simulink model "FFT4dSpace_1"  (R2021a)
settings: Solver=ode1  StartTime=0.0  StopTime=Inf  FixedStep=Ts  RelTol=1e-5
PostLoadFcn:
  | if any(exist('dsrtsu_mdlpostloadfcn', 'file') ~= 0), dsrtsu_mdlpostloadfcn('Execute', bdroot); end
InitFcn:
  | , if any(exist('rtifpga_mdlclblib', 'file') ~= 0), rtifpga_mdlclblib('Init', bdroot); end,
  | , if any(exist('dsmpb_private', 'file') ~= 0), dsmpb_private('dsmpb_mdlclblib', 'Init', bdroot); end,
values from neighbouring files (symbols this model uses):
  Ts_1kHz = 1e-3    (= 0.001)    [FFT4dSpace_1_i.m]
undefined symbols (not defined in the file or in its folder): CalibNormed, conv, mdlPara, PWMpara, Ro1_Be2, scaleHV, supplyPressure4VPPM
libraries: dsmpblib x46, tllib x2, dspxfrm3 x1, dspsigops x1
(part 2 of 2)

== system FFT4dSpace_1/RTI Data ==
  RTI Data Store : Subsystem  Tag="struct('private',struct('version',struct('dsVer',uint32(2),'dsVerCreation',uint32(2),'RTI',struct('ver','7.12','type','RTI1202')),'access',struct('type','Model','isPerm',1,'created',['29-Oct-2019 15:07:12'],'modified',['07-Feb-2024 10:56:01'],'location','')),'public',struct('main',struct('data',[]),'sub',struct('name',{{'FFT4dSpace_1'}},'data',{{struct('TH',struct('thTaskInfo',struct('taskType',{'TIMER','HWINT','TMRINT','SWINT','GLINT'},'tasksNumOf',{2,0,0,0,0},'srcIds',{{'TIMERA','TIMERA2'},{},{},{},{}},'taskNames',{{['Timer Task 1'],['Timer Task 2']},{},{},{},{}})),'th_tc',struct('dataType',{'TASK','TASK'},'taskGroupId',{'',''},'taskGroupList',{{},{}},'taskSchedulingPolicy',{'FCFS','FCFS'},'taskType',{'TIMER','TIMER'},'blkh',{-1,-1},'srcId',{'TIMERA','TIMERA2'},'srcSgnName',{['Timer A interrupt'],['Timer Task 1']},'srcCpuName',{'',''},'taskName',{['Timer Task 1  [5e-05] s'],['Timer Task 2  [0.001] s']},'taskNameDisplayExt',{'',''},'smplTime',{5e-5,0.001},'smplTimeOffs',{0,0},'hasFixedPriority',{0,0},'priority',{1,2},'hasFixedOvc',{0,0},'ovcType',{1,1},'ovcMax',{1,1}),'tc_th',struct('dataType',{'TASK','TASK'},'taskGroupId',{'',''},'taskGroupList',{{},{}},'taskSchedulingPolicy',{'FCFS','FCFS'},'taskType',{'TIMER','TIMER'},'blkh',{-1,-1},'srcId',{'TIMERA','TIMERA2'},'srcSgnName',{['Timer A interrupt'],['Timer Task 1']},'srcCpuName',{'',''},'taskName',{['Timer Task 1  [5e-05] s'],['Timer Task 2  [0.001] s']},'taskNameDisplayExt',{'',''},'smplTime',{5e-5,0.001},'smplTimeOffs',{0,0},'hasFixedPriority',{0,0},'priority',{1,2},'hasFixedOvc',{0,0},'ovcType',{1,1},'ovcMax',{1,1}),'FSIValue','0','NISValue','1')}})))"  mask(RTI_DATA_STORE){}
      mask help:
      | RTI Data Store Block. This block is used by RTI to store internal model dependent data. Deleting this block will result in data loss.
      |
      | NEVER DELETE, COPY, OR MODIFY THIS BLOCK!
      mask Help:
      | RTI Data Store Block. This block is used by RTI to store internal model dependent data. Deleting this block will result in data loss.
      | 
      | NEVER DELETE, COPY, OR MODIFY THIS BLOCK!
      mask Display: text(0.5, 0.5, ' ', 'HorizontalAlignment', 'center');

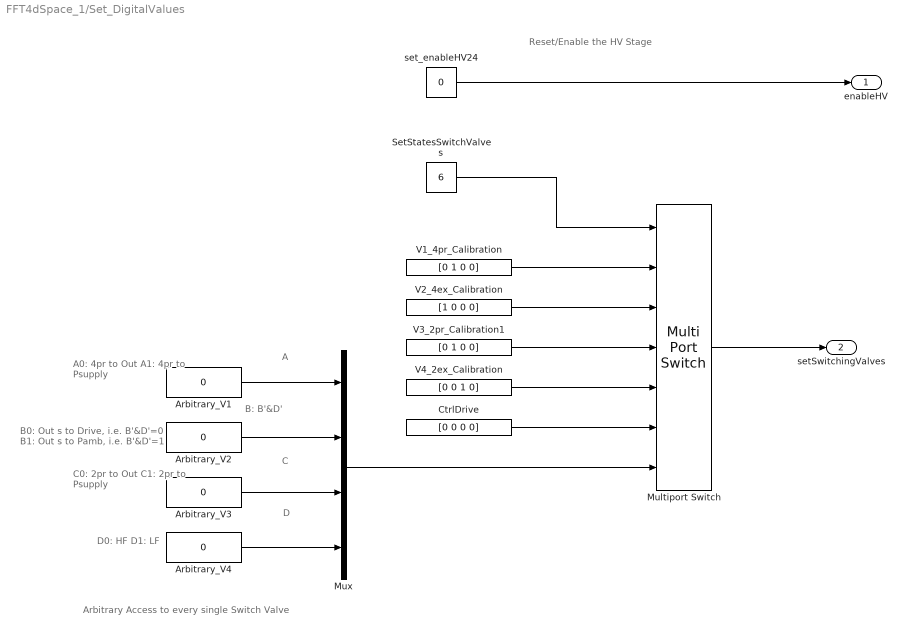
== system FFT4dSpace_1/Set_DigitalValues ==
  note: A
  note: A0: 4pr to Out
      | A1: 4pr to Psupply
  note: Arbitrary Access to every single Switch Valve
  note: Reset/Enable the HV Stage
  note: C0: 2pr to Out
      | C1: 2pr to Psupply
  note: D0: HF
      | D1: LF
  note: B0: Out s to Drive, i.e. B'&D'=0
      | B1: Out s to Pamb, i.e. B'&D'=1
  note: B: B'&D'
  note: C
  note: D
  Arbitrary_V{1..4} (4 alike) : Constant  Value=0
  CtrlDrive : Constant  Value=[0 0 0 0]  OutDataTypeStr=boolean
  Multiport Switch : MultiPortSwitch  Inputs=6
  Mux : Mux
  SetStatesSwitchValves : Constant  Value=6
  V1_4pr_Calibration : Constant  Value=[0 1 0 0]  OutDataTypeStr=boolean
  V2_4ex_Calibration : Constant  Value=[1 0 0 0]  OutDataTypeStr=boolean
  V3_2pr_Calibration1 : Constant  Value=[0 1 0 0]  OutDataTypeStr=boolean
  V4_2ex_Calibration : Constant  Value=[0 0 1 0]  OutDataTypeStr=boolean
  set_enableHV24 : Constant  Value=0  OutDataTypeStr=boolean
  "enableHV " : Outport  VectorParamsAs1DForOutWhenUnconnected=off
  setSwitchingValves : Outport  Port=2  VectorParamsAs1DForOutWhenUnconnected=off
  wires:
  SetStatesSwitchValves/1 -> Multiport Switch/1
  V1_4pr_Calibration/1 -> Multiport Switch/2
  V3_2pr_Calibration1/1 -> Multiport Switch/4
  V2_4ex_Calibration/1 -> Multiport Switch/3
  V4_2ex_Calibration/1 -> Multiport Switch/5
  CtrlDrive/1 -> Multiport Switch/6
  Mux/1 -> Multiport Switch/7
  Multiport Switch/1 -> setSwitchingValves/1
  set_enableHV24/1 -> "enableHV "/1
  Arbitrary_V2/1 -> Mux/2
  Arbitrary_V4/1 -> Mux/4
  Arbitrary_V3/1 -> Mux/3
  Arbitrary_V1/1 -> Mux/1

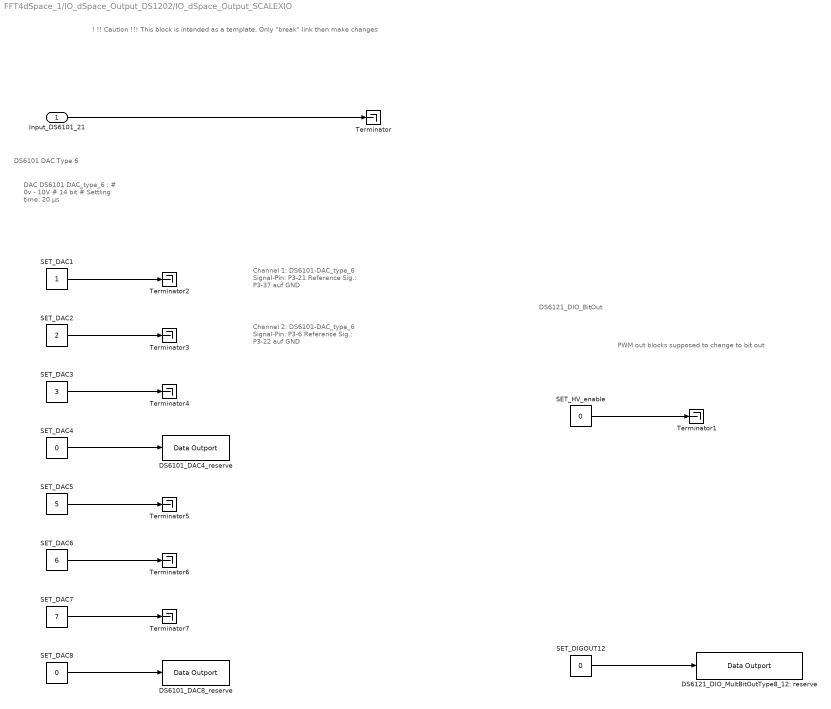
== system FFT4dSpace_1/IO_dSpace_Output_DS1202/IO_dSpace_Output_SCALEXIO ==
  note: PWM out blocks supposed to change to bit out
  note: DS6121_DIO_BitOut
  note: Channel 1: DS6101-DAC_type_6
      | Signal-Pin: P3-21
      | Reference Sig.: P3-37 auf GND
  note: DS6101 DAC Type 6
  note: Channel 2: DS6101-DAC_type_6
      | Signal-Pin: P3-6
      | Reference Sig.: P3-22 auf GND
  note: DAC DS6101 DAC_type_6 :
      | # 0v - 10V
      | # 14 bit
      | # Settling time: 20 µs
  note: ! !! Caution !!!
      | This block is intended as a template.
      | Only "break" link then make changes
  Input_DS6101_21 : Inport
  DS6101_DAC4_reserve : dsmpblib/Data Outport  Priority=-10000
      settings: SourceProductName=dSPACE Model Interface Blockset
  DS6101_DAC8_reserve : dsmpblib/Data Outport  Priority=-10000
      settings: SourceProductName=dSPACE Model Interface Blockset
  DS6121_DIO_MultBitOutType8_12: reserve : dsmpblib/Data Outport  Priority=-10000
      settings: SourceProductName=dSPACE Model Interface Blockset
  SET_DAC1 : Constant
  SET_DAC2 : Constant  Value=2
  SET_DAC3 : Constant  Value=3
  SET_DAC4 : Constant  Value=0
  SET_DAC5 : Constant  Value=5
  SET_DAC6 : Constant  Value=6
  SET_DAC7 : Constant  Value=7
  SET_DAC8 : Constant  Value=0
  SET_DIGOUT12 : Constant  Value=0  OutDataTypeStr=boolean
  SET_HV_enable : Constant  Value=0  OutDataTypeStr=boolean
  Terminator{,1..7} (8 alike) : Terminator
  wires:
  SET_DAC1/1 -> Terminator2/1
  Input_DS6101_21/1 -> Terminator/1
  SET_DAC2/1 -> Terminator3/1
  SET_DAC4/1 -> DS6101_DAC4_reserve/1
  SET_DAC3/1 -> Terminator4/1
  SET_DAC6/1 -> Terminator6/1
  SET_DAC5/1 -> Terminator5/1
  SET_DAC7/1 -> Terminator7/1
  SET_DAC8/1 -> DS6101_DAC8_reserve/1
  SET_HV_enable/1 -> Terminator1/1
  SET_DIGOUT12/1 -> DS6121_DIO_MultBitOutType8_12: reserve/1

== system FFT4dSpace_1/IO_dSpace_Output_DS1202/PWMcompNegativ ==
  In1 : Inport
  Add1 : Sum
  Constant1 : Constant  Value=0
  Constant2 : Constant  Value=PWMpara.offsetNegativ
  Switch : Switch  Criteria=u2 > Threshold  Threshold=PWMpara.thresholdNegativ
  PWMplusNegativ : Outport
  wires:
  Constant1/1 -> Switch/3
  Switch/1 -> Add1/1
  Constant2/1 -> Switch/1
  Add1/1 -> PWMplusNegativ/1  "PWMplusNegativ"
  In1/1 -> Add1/2, Switch/2

== system FFT4dSpace_1/IO_dSpace_Output_DS1202/PWMcompPositiv ==
  In1 : Inport
  Add1 : Sum
  Constant1 : Constant  Value=0
  Constant2 : Constant  Value=PWMpara.offsetPositiv
  Switch : Switch  Criteria=u2 > Threshold  Threshold=PWMpara.thresholdPositiv
  PWMplusPositiv : Outport
  wires:
  Constant1/1 -> Switch/3
  Switch/1 -> Add1/1
  Constant2/1 -> Switch/1
  Add1/1 -> PWMplusPositiv/1  "PWMplusPositiv"
  In1/1 -> Add1/2, Switch/2

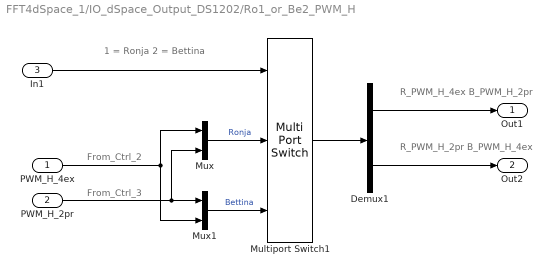
== system FFT4dSpace_1/IO_dSpace_Output_DS1202/Ro1_or_Be2_PWM_H ==
  note: 1 = Ronja
      | 2 = Bettina
  note: From_Ctrl_2
  note: R_PWM_H_4ex
      | B_PWM_H_2pr
  note: R_PWM_H_2pr
      | B_PWM_H_4ex
  note: From_Ctrl_3
  PWM_H_4ex : Inport
  PWM_H_2pr : Inport  Port=2
  In1 : Inport  Port=3
  Demux1 : Demux  Outputs=2
  Multiport Switch1 : MultiPortSwitch  Inputs=2
  Mux : Mux  Inputs=2
  Mux1 : Mux  Inputs=2
  Out1 : Outport
  Out2 : Outport  Port=2
  wires:
  Mux1/1 -> Multiport Switch1/3  "Bettina"
  Mux/1 -> Multiport Switch1/2  "Ronja"
  PWM_H_2pr/1 -> Mux/2, Mux1/1
  Multiport Switch1/1 -> Demux1/1
  Demux1/1 -> Out1/1
  PWM_H_4ex/1 -> Mux/1, Mux1/2
  Demux1/2 -> Out2/1
  In1/1 -> Multiport Switch1/1

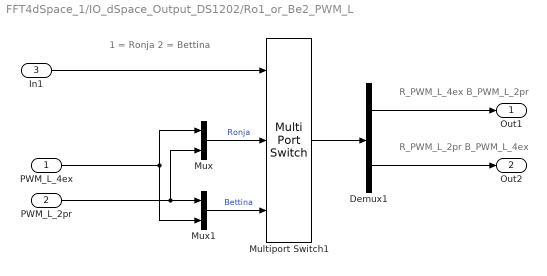
== system FFT4dSpace_1/IO_dSpace_Output_DS1202/Ro1_or_Be2_PWM_L ==
  note: R_PWM_L_4ex
      | B_PWM_L_2pr
  note: R_PWM_L_2pr
      | B_PWM_L_4ex
  note: 1 = Ronja
      | 2 = Bettina
  PWM_L_4ex : Inport
  PWM_L_2pr : Inport  Port=2
  In1 : Inport  Port=3
  Demux1 : Demux  Outputs=2
  Multiport Switch1 : MultiPortSwitch  Inputs=2
  Mux : Mux  Inputs=2
  Mux1 : Mux  Inputs=2
  Out1 : Outport
  Out2 : Outport  Port=2
  wires:
  Mux1/1 -> Multiport Switch1/3  "Bettina"
  Mux/1 -> Multiport Switch1/2  "Ronja"
  PWM_L_2pr/1 -> Mux/2, Mux1/1
  Multiport Switch1/1 -> Demux1/1
  Demux1/1 -> Out1/1
  PWM_L_4ex/1 -> Mux/1, Mux1/2
  Demux1/2 -> Out2/1
  In1/1 -> Multiport Switch1/1

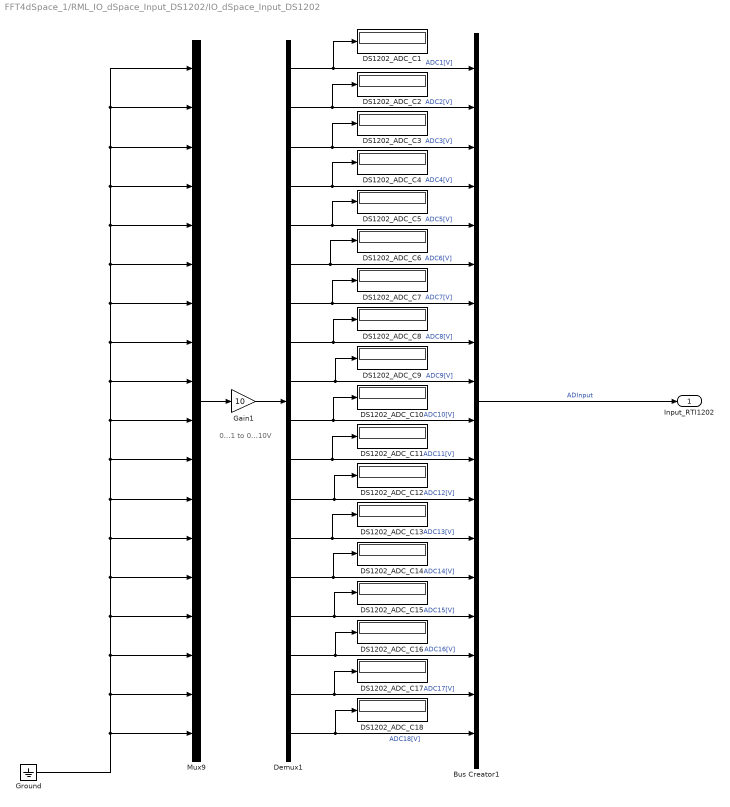
== system FFT4dSpace_1/RML_IO_dSpace_Input_DS1202/IO_dSpace_Input_DS1202 ==
  note: 0...1 to 0...10V
  Bus Creator1 : BusCreator  Inputs=18
  DS1202_ADC_C{1..18} (18 alike) : Display
  Demux1 : Demux  Outputs=18
  Gain1 : Gain  Gain=10
  Ground : Ground
  Mux9 : Mux  Inputs=18
  Input_RTI1202 : Outport
  wires:
  Gain1/1 -> Demux1/1
  Mux9/1 -> Gain1/1
  Demux1/16 -> DS1202_ADC_C16/1, Bus Creator1/16  "ADC16[V]"
  Demux1/15 -> DS1202_ADC_C15/1, Bus Creator1/15  "ADC15[V]"
  Demux1/14 -> DS1202_ADC_C14/1, Bus Creator1/14  "ADC14[V]"
  Demux1/13 -> DS1202_ADC_C13/1, Bus Creator1/13  "ADC13[V]"
  Demux1/12 -> DS1202_ADC_C12/1, Bus Creator1/12  "ADC12[V]"
  Demux1/11 -> DS1202_ADC_C11/1, Bus Creator1/11  "ADC11[V]"
  Demux1/10 -> DS1202_ADC_C10/1, Bus Creator1/10  "ADC10[V]"
  Demux1/9 -> Bus Creator1/9, DS1202_ADC_C9/1  "ADC9[V]"
  Demux1/8 -> DS1202_ADC_C8/1, Bus Creator1/8  "ADC8[V]"
  Demux1/7 -> DS1202_ADC_C7/1, Bus Creator1/7  "ADC7[V]"
  Demux1/6 -> DS1202_ADC_C6/1, Bus Creator1/6  "ADC6[V]"
  Demux1/5 -> DS1202_ADC_C5/1, Bus Creator1/5  "ADC5[V]"
  Demux1/4 -> DS1202_ADC_C4/1, Bus Creator1/4  "ADC4[V]"
  Demux1/3 -> DS1202_ADC_C3/1, Bus Creator1/3  "ADC3[V]"
  Demux1/2 -> DS1202_ADC_C2/1, Bus Creator1/2  "ADC2[V]"
  Demux1/1 -> DS1202_ADC_C1/1, Bus Creator1/1  "ADC1[V]"
  Bus Creator1/1 -> Input_RTI1202/1  "ADInput"
  Demux1/17 -> DS1202_ADC_C17/1, Bus Creator1/17  "ADC17[V]"
  Demux1/18 -> Bus Creator1/18, DS1202_ADC_C18/1  "ADC18[V]"
  Ground/1 -> Mux9/18, Mux9/17, Mux9/16, Mux9/15, Mux9/14, Mux9/13, Mux9/12, Mux9/11, Mux9/10, Mux9/9, Mux9/8, Mux9/7, Mux9/6, Mux9/5, Mux9/4, Mux9/3, Mux9/2, Mux9/1

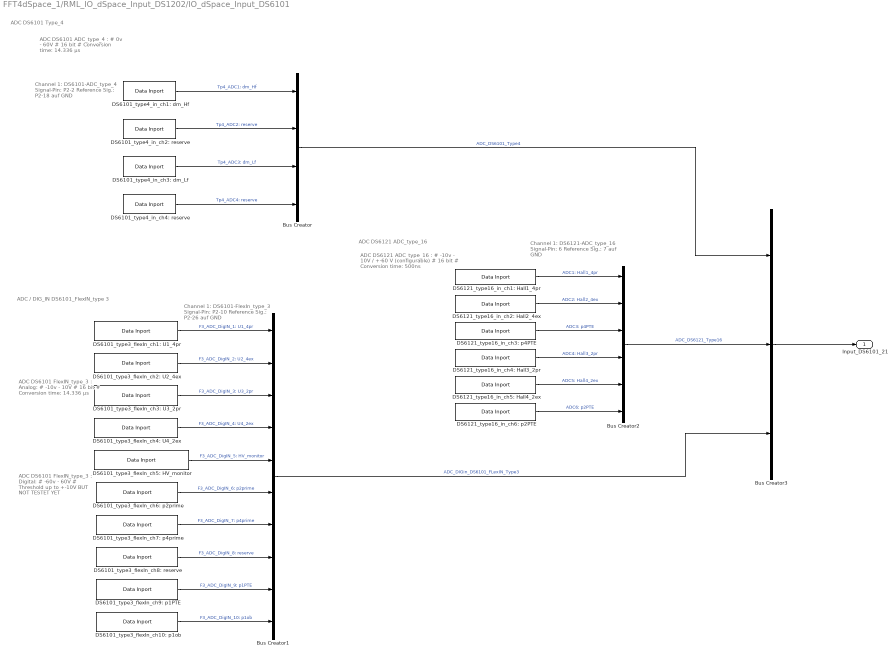
== system FFT4dSpace_1/RML_IO_dSpace_Input_DS1202/IO_dSpace_Input_DS6101 ==
  note: ADC / DIG_IN DS6101_FlexIN_type 3
  note: ADC DS6101 Type_4
  note: ADC DS6121 ADC_type_16
  note: Channel 1: DS6101-ADC_type_4
      | Signal-Pin: P2-2
      | Reference Sig.: P2-18 auf GND
  note: ADC DS6101 ADC_type_4 :
      | # 0v - 60V
      | # 16 bit
      | # Conversion time: 14.336 µs
  note: Channel 1: DS6101-FlexIn_type_3
      | Signal-Pin: P2-10
      | Reference Sig.: P2-26 auf GND
  note: ADC DS6101 FlexIN_type_3 :
      | Analog:
      | # -10v - 10V
      | # 16 bit
      | # Conversion time: 14.336 µs
  note: ADC DS6101 FlexIN_type_3 :
      | Digital:
      | # -60v - 60V
      | # Threshold up to +-10V
      |
      | BUT NOT TESTET YET
  note: Channel 1: DS6121-ADC_type_16
      | Signal-Pin: 6
      | Reference Sig.: 7 auf GND
  note: ADC DS6121 ADC_type_16 :
      | # -10v - 10V / +-60 V (configurable)
      | # 16 bit
      | # Conversion time: 500ns
  Bus Creator : BusCreator  Inputs=4
  Bus Creator1 : BusCreator  Inputs=10
  Bus Creator2 : BusCreator  Inputs=6
  Bus Creator3 : BusCreator  Inputs=3
  DS6101_type3_flexIn_ch10: p1ob : dsmpblib/Data Inport  Priority=10000
      settings: SourceProductName=dSPACE Model Interface Blockset
  DS6101_type3_flexIn_ch1: U1_4pr : dsmpblib/Data Inport  Priority=10000
      settings: SourceProductName=dSPACE Model Interface Blockset
  "DS6101_type3_flexIn_ch2: U2_4ex " : dsmpblib/Data Inport  Priority=10000
      settings: SourceProductName=dSPACE Model Interface Blockset
  DS6101_type3_flexIn_ch3: U3_2pr : dsmpblib/Data Inport  Priority=10000
      settings: SourceProductName=dSPACE Model Interface Blockset
  DS6101_type3_flexIn_ch4: U4_2ex : dsmpblib/Data Inport  Priority=10000
      settings: SourceProductName=dSPACE Model Interface Blockset
  DS6101_type3_flexIn_ch5: HV_monitor : dsmpblib/Data Inport  Priority=10000
      settings: SourceProductName=dSPACE Model Interface Blockset
  DS6101_type3_flexIn_ch6: p2prime : dsmpblib/Data Inport  Priority=10000
      settings: SourceProductName=dSPACE Model Interface Blockset
  DS6101_type3_flexIn_ch7: p4prime : dsmpblib/Data Inport  Priority=10000
      settings: SourceProductName=dSPACE Model Interface Blockset
  DS6101_type3_flexIn_ch8: reserve : dsmpblib/Data Inport  Priority=10000
      settings: SourceProductName=dSPACE Model Interface Blockset
  DS6101_type3_flexIn_ch9: p1PTE : dsmpblib/Data Inport  Priority=10000
      settings: SourceProductName=dSPACE Model Interface Blockset
  DS6101_type4_in_ch1: dm_Hf : dsmpblib/Data Inport  Priority=10000
      settings: SourceProductName=dSPACE Model Interface Blockset
  DS6101_type4_in_ch2: reserve : dsmpblib/Data Inport  Priority=10000
      settings: SourceProductName=dSPACE Model Interface Blockset
  DS6101_type4_in_ch3: dm_Lf : dsmpblib/Data Inport  Priority=10000
      settings: SourceProductName=dSPACE Model Interface Blockset
  DS6101_type4_in_ch4: reserve : dsmpblib/Data Inport  Priority=10000
      settings: SourceProductName=dSPACE Model Interface Blockset
  DS6121_type16_in_ch1: Hall1_4pr : dsmpblib/Data Inport  Priority=10000
      settings: SourceProductName=dSPACE Model Interface Blockset
  DS6121_type16_in_ch2: Hall2_4ex : dsmpblib/Data Inport  Priority=10000
      settings: SourceProductName=dSPACE Model Interface Blockset
  DS6121_type16_in_ch3: p4PTE : dsmpblib/Data Inport  Priority=10000
      settings: SourceProductName=dSPACE Model Interface Blockset
  DS6121_type16_in_ch4: Hall3_2pr : dsmpblib/Data Inport  Priority=10000
      settings: SourceProductName=dSPACE Model Interface Blockset
  DS6121_type16_in_ch5: Hall4_2ex : dsmpblib/Data Inport  Priority=10000
      settings: SourceProductName=dSPACE Model Interface Blockset
  DS6121_type16_in_ch6: p2PTE : dsmpblib/Data Inport  Priority=10000
      settings: SourceProductName=dSPACE Model Interface Blockset
  Input_DS6101_21 : Outport
  wires:
  "DS6101_type3_flexIn_ch2: U2_4ex "/1 -> Bus Creator1/2  "F3_ADC_DigIN_2: U2_4ex"
  DS6121_type16_in_ch1: Hall1_4pr/1 -> Bus Creator2/1  "ADC1: Hall1_4pr"
  DS6101_type4_in_ch1: dm_Hf/1 -> Bus Creator/1  "Tp4_ADC1: dm_Hf"
  DS6101_type4_in_ch2: reserve/1 -> Bus Creator/2  "Tp4_ADC2: reserve"
  DS6101_type4_in_ch3: dm_Lf/1 -> Bus Creator/3  "Tp4_ADC3: dm_Lf"
  DS6101_type4_in_ch4: reserve/1 -> Bus Creator/4  "Tp4_ADC4: reserve"
  Bus Creator/1 -> Bus Creator3/1  "ADC_DS6101_Type4"
  DS6101_type3_flexIn_ch1: U1_4pr/1 -> Bus Creator1/1  "F3_ADC_DigIN_1: U1_4pr"
  DS6101_type3_flexIn_ch3: U3_2pr/1 -> Bus Creator1/3  "F3_ADC_DigIN_3: U3_2pr"
  DS6101_type3_flexIn_ch4: U4_2ex/1 -> Bus Creator1/4  "F3_ADC_DigIN_4: U4_2ex"
  DS6101_type3_flexIn_ch7: p4prime/1 -> Bus Creator1/7  "F3_ADC_DigIN_7: p4prime"
  DS6101_type3_flexIn_ch5: HV_monitor/1 -> Bus Creator1/5  "F3_ADC_DigIN_5: HV_monitor"
  DS6101_type3_flexIn_ch8: reserve/1 -> Bus Creator1/8  "F3_ADC_DigIN_8: reserve"
  DS6101_type3_flexIn_ch6: p2prime/1 -> Bus Creator1/6  "F3_ADC_DigIN_6: p2prime"
  DS6101_type3_flexIn_ch10: p1ob/1 -> Bus Creator1/10  "F3_ADC_DigIN_10: p1ob"
  DS6101_type3_flexIn_ch9: p1PTE/1 -> Bus Creator1/9  "F3_ADC_DigIN_9: p1PTE"
  DS6121_type16_in_ch2: Hall2_4ex/1 -> Bus Creator2/2  "ADC2: Hall2_4ex"
  DS6121_type16_in_ch4: Hall3_2pr/1 -> Bus Creator2/4  "ADC4: Hall3_2pr"
  DS6121_type16_in_ch3: p4PTE/1 -> Bus Creator2/3  "ADC3: p4PTE"
  Bus Creator3/1 -> Input_DS6101_21/1
  DS6121_type16_in_ch6: p2PTE/1 -> Bus Creator2/6  "ADC6: p2PTE"
  DS6121_type16_in_ch5: Hall4_2ex/1 -> Bus Creator2/5  "ADC5: Hall4_2ex"
  Bus Creator2/1 -> Bus Creator3/2  "ADC_DS6121_Type16"
  Bus Creator1/1 -> Bus Creator3/3  "ADC_DIGin_DS6101_FLexIN_Type3"

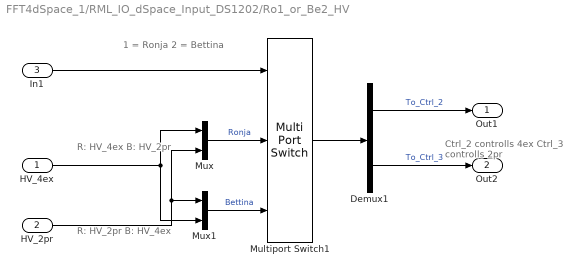
== system FFT4dSpace_1/RML_IO_dSpace_Input_DS1202/Ro1_or_Be2_HV ==
  note: Ctrl_2 controlls 4ex
      | Ctrl_3 controlls 2pr
  note: 1 = Ronja
      | 2 = Bettina
  note: R: HV_4ex
      | B: HV_2pr
  note: R: HV_2pr
      | B: HV_4ex
  HV_4ex : Inport
  HV_2pr : Inport  Port=2
  In1 : Inport  Port=3
  Demux1 : Demux  Outputs=2
  Multiport Switch1 : MultiPortSwitch  Inputs=2
  Mux : Mux  Inputs=2
  Mux1 : Mux  Inputs=2
  Out1 : Outport
  Out2 : Outport  Port=2
  wires:
  Mux1/1 -> Multiport Switch1/3  "Bettina"
  Mux/1 -> Multiport Switch1/2  "Ronja"
  HV_2pr/1 -> Mux/2, Mux1/1
  Multiport Switch1/1 -> Demux1/1
  Demux1/1 -> Out1/1  "To_Ctrl_2"
  HV_4ex/1 -> Mux1/2, Mux/1
  Demux1/2 -> Out2/1  "To_Ctrl_3"
  In1/1 -> Multiport Switch1/1

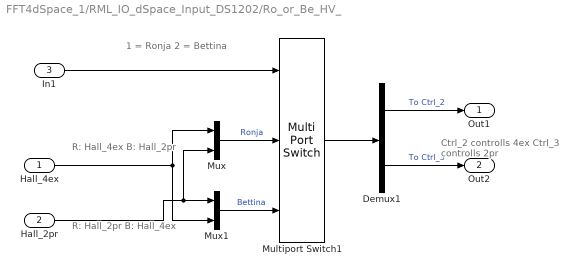
== system FFT4dSpace_1/RML_IO_dSpace_Input_DS1202/Ro_or_Be_HV_ ==
  note: Ctrl_2 controlls 4ex
      | Ctrl_3 controlls 2pr
  note: 1 = Ronja
      | 2 = Bettina
  note: R: Hall_4ex
      | B: Hall_2pr
  note: R: Hall_2pr
      | B: Hall_4ex
  Hall_4ex : Inport
  Hall_2pr : Inport  Port=2
  In1 : Inport  Port=3
  Demux1 : Demux  Outputs=2
  Multiport Switch1 : MultiPortSwitch  Inputs=2
  Mux : Mux  Inputs=2
  Mux1 : Mux  Inputs=2
  Out1 : Outport
  Out2 : Outport  Port=2
  wires:
  In1/1 -> Multiport Switch1/1
  Demux1/2 -> Out2/1  "To Ctrl_3"
  Hall_4ex/1 -> Mux1/2, Mux/1
  Demux1/1 -> Out1/1  "To Ctrl_2"
  Multiport Switch1/1 -> Demux1/1
  Hall_2pr/1 -> Mux1/1, Mux/2
  Mux/1 -> Multiport Switch1/2  "Ronja"
  Mux1/1 -> Multiport Switch1/3  "Bettina"

== system FFT4dSpace_1/RTI Data/RTI Data Store ==
  RTI Data Store : Subsystem  mask(RTI_DATA_STORE){}
      mask help:
      | RTI Data Store Block. This block is used by RTI to store internal model dependent data. Deleting this block will result in data loss.
      |
      | NEVER DELETE, COPY, OR MODIFY THIS BLOCK!
      mask Help:
      | RTI Data Store Block. This block is used by RTI to store internal model dependent data. Deleting this block will result in data loss.
      | 
      | NEVER DELETE, COPY, OR MODIFY THIS BLOCK!
      mask Display: text(0.5, 0.5, ' ', 'HorizontalAlignment', 'center');

== system FFT4dSpace_1/RTI Data/RTI Data Store/RTI Data Store ==
  RTI Data Store : Subsystem  mask(RTI_DATA_STORE){}
      mask help:
      | RTI Data Store Block. This block is used by RTI to store internal model dependent data. Deleting this block will result in data loss.
      |
      | NEVER DELETE, COPY, OR MODIFY THIS BLOCK!
      mask Help:
      | RTI Data Store Block. This block is used by RTI to store internal model dependent data. Deleting this block will result in data loss.
      | 
      | NEVER DELETE, COPY, OR MODIFY THIS BLOCK!
      mask Display: text(0.5, 0.5, ' ', 'HorizontalAlignment', 'center');

== system FFT4dSpace_1/RTI Data/RTI Data Store/RTI Data Store/RTI Data Store ==
  RTI Data Store : Subsystem  mask(RTI_DATA_STORE){}
      mask help:
      | RTI Data Store Block. This block is used by RTI to store internal model dependent data. Deleting this block will result in data loss.
      |
      | NEVER DELETE, COPY, OR MODIFY THIS BLOCK!
      mask Help:
      | RTI Data Store Block. This block is used by RTI to store internal model dependent data. Deleting this block will result in data loss.
      | 
      | NEVER DELETE, COPY, OR MODIFY THIS BLOCK!
      mask Display: text(0.5, 0.5, ' ', 'HorizontalAlignment', 'center');

== system FFT4dSpace_1/RTI Data/RTI Data Store/RTI Data Store/RTI Data Store/RTI Data Store ==

== matlab function FFT4dSpace_1/RML_IO_dSpace_Input_DS1202/Hall_To_Prc1 ==
  data: Udn input; Vout output; Uup input; Vdn input; Vup input; HallSignal input; lambda output
function [Vout, lambda] = fcn(Udn,Uup,Vdn,Vup,HallSignal)
    m = (Vup-Vdn)/(Uup - Udn);
    c = Vup - m*Uup ;
Vout = m*HallSignal + c;
lambda = m; %Slope [(nL/min)/V] [nL/(min V)]

== matlab function FFT4dSpace_1/RML_IO_dSpace_Input_DS1202/Hall_To_Prc2 ==
  data: Udn input; Vout output; Uup input; Vdn input; Vup input; HallSignal input; lambda output
function [Vout, lambda] = fcn(Udn,Uup,Vdn,Vup,HallSignal)
    m = (Vup-Vdn)/(Uup - Udn);
    c = Vup - m*Uup ;
Vout = m*HallSignal + c;
lambda = m; %Slope [(nL/min)/V] [nL/(min V)]

== matlab function FFT4dSpace_1/RML_IO_dSpace_Input_DS1202/Hall_To_Prc3 ==
  data: Udn input; Vout output; Uup input; Vdn input; Vup input; HallSignal input; lambda output
function [Vout, lambda] = fcn(Udn,Uup,Vdn,Vup,HallSignal)
    m = (Vup-Vdn)/(Uup - Udn);
    c = Vup - m*Uup ;
Vout = m*HallSignal + c;
lambda = m; %Slope [(nL/min)/V] [nL/(min V)]

== matlab function FFT4dSpace_1/RML_IO_dSpace_Input_DS1202/Hall_To_Prc4 ==
  data: Udn input; Vout output; Uup input; Vdn input; Vup input; HallSignal input; lambda output
function [Vout, lambda] = fcn(Udn,Uup,Vdn,Vup,HallSignal)
    m = (Vup-Vdn)/(Uup - Udn);
    c = Vup - m*Uup ;
Vout = m*HallSignal + c;
lambda = m; %Slope [(nL/min)/V] [nL/(min V)]

== matlab function FFT4dSpace_1/RML_IO_dSpace_Input_DS1202/Compute_delta_percent ==
  data: deltaVec input; deltaPercentVec output; lambdaVec input; VmaxVec input
function deltaPercentVec  = fcn(deltaVec,lambdaVec,VmaxVec)
% Calculating the deltas in % out of measured deltas in V
% ** delta_% = delta_V*lambda/Vmax **

% 11.08.2023, nitr
deltaPercentVec = deltaVec.*lambdaVec./VmaxVec*100; % [%]

== matlab function FFT4dSpace_1/MATLAB Function1 ==
  data: myTime input; y_sin output; compFreq_Hz input; compPhase_deg input
function y_sin  = fcn(myTime,compFreq_Hz,compPhase_deg)
% Computation of a sinus to compensate the squeazing vibrations actively
y_sin = sin(myTime*compFreq_Hz*2*pi + compPhase_deg*pi/180)
% y = u;
